simulink model "Golf_Lin_Modale"  (R2019a)
settings: Solver=VariableStepAuto  StartTime=0.0  StopTime=7  RelTol=1e-3
undefined symbols (not defined in the file or in its folder): A6, B6, C6, Cobs, H, K_i, K_x, L6
settings Model: Creator=ulyss  LastModifiedBy=mariu

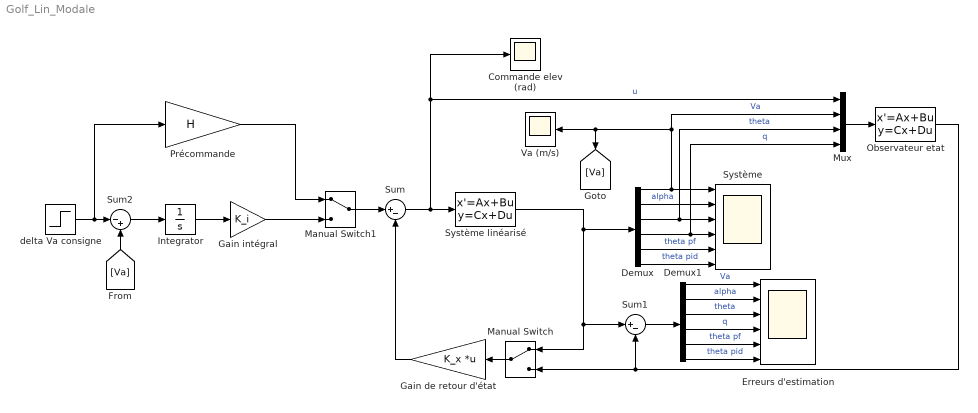
== system Golf_Lin_Modale ==
  Commande elev (rad) : Scope
  Demux : Demux  Outputs=6
  Demux1 : Demux  Outputs=6
  Erreurs d'estimation : Scope  NumInputPorts=6
  Gain de retour d'état : Gain  Gain=K_x  Multiplication=Matrix(K*u) (u vector)
  Gain intégral : Gain  Gain=K_i
  Integrator : Integrator
  Manual Switch : ManualSwitch
  Manual Switch1 : ManualSwitch
  Mux : Mux
  Observateur etat : StateSpace  A=A6-L6*Cobs  B=[B6, L6]  C=eye(6)  D=zeros(6,4)  InitialCondition=0
  Précommande : Gain  Gain=H
  Sum : Sum  Inputs=|+-
  Sum1 : Sum  Inputs=|+-
  Sum2 : Sum  Inputs=|-+
  Système : Scope  NumInputPorts=6
  Système linéarisé : StateSpace  A=A6  B=B6  C=C6  D=zeros(6,1)  InitialCondition=rand(6,1)
  Va (m/s) : Scope
  delta Va consigne : Step  After=3  SampleTime=0
  wires:
  Sum/1 -> Commande elev (rad)/1, Mux/1, Système linéarisé/1  "u"
  Système linéarisé/1 -> Demux/1, Manual Switch/1, Sum1/1
  Gain de retour d'état/1 -> Sum/2
  delta Va consigne/1 -> Précommande/1, Sum2/1
  Demux/1 -> Mux/2, [Va], Va (m/s)/1, Système/1  "Va"
  Demux/2 -> Système/2  "alpha"
  Demux/5 -> Système/5  "theta pf"
  Demux/6 -> Système/6  "theta pid"
  Demux/3 -> Système/3, Mux/3  "theta"
  Demux/4 -> Mux/4, Système/4  "q"
  Manual Switch/1 -> Gain de retour d'état/1
  Observateur etat/1 -> Manual Switch/2, Sum1/2
  Mux/1 -> Observateur etat/1
  Précommande/1 -> Manual Switch1/1
  Manual Switch1/1 -> Sum/1
  [Va] -> Sum2/2
  Sum2/1 -> Integrator/1
  Integrator/1 -> Gain intégral/1
  Gain intégral/1 -> Manual Switch1/2
  Sum1/1 -> Demux1/1
  Demux1/1 -> Erreurs d'estimation/1  "Va"
  Demux1/5 -> Erreurs d'estimation/5  "theta pf"
  Demux1/3 -> Erreurs d'estimation/3  "theta"
  Demux1/2 -> Erreurs d'estimation/2  "alpha"
  Demux1/6 -> Erreurs d'estimation/6  "theta pid"
  Demux1/4 -> Erreurs d'estimation/4  "q"
